simulink model "sevietta_devel_2018a"  (R2013a)
settings: Solver=VariableStepDiscrete  SolverMode=SingleTasking  StartTime=0.0  StopTime=3276  RelTol=1e-3
undefined symbols (not defined in the file): sfp
libraries: xbsIndex_r4 x2589, casper_library_delays x40, simulink x19, casper_library_misc x17, xps_library x13
(part 7 of 32)

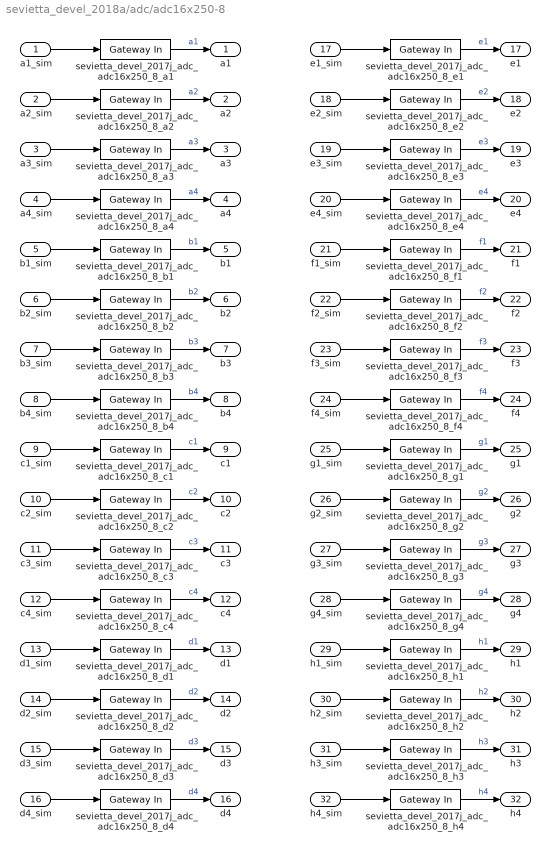
== system sevietta_devel_2018a/adc/adc16x250-8 ==
  a1_sim : Inport
  a2_sim : Inport  Port=2
  a3_sim : Inport  Port=3
  a4_sim : Inport  Port=4
  b1_sim : Inport  Port=5
  b2_sim : Inport  Port=6
  b3_sim : Inport  Port=7
  b4_sim : Inport  Port=8
  c1_sim : Inport  Port=9
  c2_sim : Inport  Port=10
  c3_sim : Inport  Port=11
  c4_sim : Inport  Port=12
  d1_sim : Inport  Port=13
  d2_sim : Inport  Port=14
  d3_sim : Inport  Port=15
  d4_sim : Inport  Port=16
  e1_sim : Inport  Port=17
  e2_sim : Inport  Port=18
  e3_sim : Inport  Port=19
  e4_sim : Inport  Port=20
  f1_sim : Inport  Port=21
  f2_sim : Inport  Port=22
  f3_sim : Inport  Port=23
  f4_sim : Inport  Port=24
  g1_sim : Inport  Port=25
  g2_sim : Inport  Port=26
  g3_sim : Inport  Port=27
  g4_sim : Inport  Port=28
  h1_sim : Inport  Port=29
  h2_sim : Inport  Port=30
  h3_sim : Inport  Port=31
  h4_sim : Inport  Port=32
  sevietta_devel_2017j_adc_adc16x250_8_a{1..4} (4 alike) : xbsIndex_r4/Gateway In  gui_display_data_type=Fixed-point  arith_type="Signed  (2's comp)"  n_bits=8  bin_pt=7  preci_type=Single  exp_width=8  frac_width=24  quantization="Round  (unbiased: +/- Inf)"  overflow=Saturate  period=1  dbl_ovrd=off  timing_constraint=None  locs_specified=off  LOCs={}  UseAsADC=off  ADCChannel='1'  inherit_from_input=off  hdl_port=on  block_type=gatewayin
  sevietta_devel_2017j_adc_adc16x250_8_b{1..4} (4 alike) : xbsIndex_r4/Gateway In  gui_display_data_type=Fixed-point  arith_type="Signed  (2's comp)"  n_bits=8  bin_pt=7  preci_type=Single  exp_width=8  frac_width=24  quantization="Round  (unbiased: +/- Inf)"  overflow=Saturate  period=1  dbl_ovrd=off  timing_constraint=None  locs_specified=off  LOCs={}  UseAsADC=off  ADCChannel='1'  inherit_from_input=off  hdl_port=on  block_type=gatewayin
  sevietta_devel_2017j_adc_adc16x250_8_c{1..4} (4 alike) : xbsIndex_r4/Gateway In  gui_display_data_type=Fixed-point  arith_type="Signed  (2's comp)"  n_bits=8  bin_pt=7  preci_type=Single  exp_width=8  frac_width=24  quantization="Round  (unbiased: +/- Inf)"  overflow=Saturate  period=1  dbl_ovrd=off  timing_constraint=None  locs_specified=off  LOCs={}  UseAsADC=off  ADCChannel='1'  inherit_from_input=off  hdl_port=on  block_type=gatewayin
  sevietta_devel_2017j_adc_adc16x250_8_d{1..4} (4 alike) : xbsIndex_r4/Gateway In  gui_display_data_type=Fixed-point  arith_type="Signed  (2's comp)"  n_bits=8  bin_pt=7  preci_type=Single  exp_width=8  frac_width=24  quantization="Round  (unbiased: +/- Inf)"  overflow=Saturate  period=1  dbl_ovrd=off  timing_constraint=None  locs_specified=off  LOCs={}  UseAsADC=off  ADCChannel='1'  inherit_from_input=off  hdl_port=on  block_type=gatewayin
  sevietta_devel_2017j_adc_adc16x250_8_e{1..4} (4 alike) : xbsIndex_r4/Gateway In  gui_display_data_type=Fixed-point  arith_type="Signed  (2's comp)"  n_bits=8  bin_pt=7  preci_type=Single  exp_width=8  frac_width=24  quantization="Round  (unbiased: +/- Inf)"  overflow=Saturate  period=1  dbl_ovrd=off  timing_constraint=None  locs_specified=off  LOCs={}  UseAsADC=off  ADCChannel='1'  inherit_from_input=off  hdl_port=on  block_type=gatewayin
  sevietta_devel_2017j_adc_adc16x250_8_f{1..4} (4 alike) : xbsIndex_r4/Gateway In  gui_display_data_type=Fixed-point  arith_type="Signed  (2's comp)"  n_bits=8  bin_pt=7  preci_type=Single  exp_width=8  frac_width=24  quantization="Round  (unbiased: +/- Inf)"  overflow=Saturate  period=1  dbl_ovrd=off  timing_constraint=None  locs_specified=off  LOCs={}  UseAsADC=off  ADCChannel='1'  inherit_from_input=off  hdl_port=on  block_type=gatewayin
  sevietta_devel_2017j_adc_adc16x250_8_g{1..4} (4 alike) : xbsIndex_r4/Gateway In  gui_display_data_type=Fixed-point  arith_type="Signed  (2's comp)"  n_bits=8  bin_pt=7  preci_type=Single  exp_width=8  frac_width=24  quantization="Round  (unbiased: +/- Inf)"  overflow=Saturate  period=1  dbl_ovrd=off  timing_constraint=None  locs_specified=off  LOCs={}  UseAsADC=off  ADCChannel='1'  inherit_from_input=off  hdl_port=on  block_type=gatewayin
  sevietta_devel_2017j_adc_adc16x250_8_h{1..4} (4 alike) : xbsIndex_r4/Gateway In  gui_display_data_type=Fixed-point  arith_type="Signed  (2's comp)"  n_bits=8  bin_pt=7  preci_type=Single  exp_width=8  frac_width=24  quantization="Round  (unbiased: +/- Inf)"  overflow=Saturate  period=1  dbl_ovrd=off  timing_constraint=None  locs_specified=off  LOCs={}  UseAsADC=off  ADCChannel='1'  inherit_from_input=off  hdl_port=on  block_type=gatewayin
  a1 : Outport
  a2 : Outport  Port=2
  a3 : Outport  Port=3
  a4 : Outport  Port=4
  b1 : Outport  Port=5
  b2 : Outport  Port=6
  b3 : Outport  Port=7
  b4 : Outport  Port=8
  c1 : Outport  Port=9
  c2 : Outport  Port=10
  c3 : Outport  Port=11
  c4 : Outport  Port=12
  d1 : Outport  Port=13
  d2 : Outport  Port=14
  d3 : Outport  Port=15
  d4 : Outport  Port=16
  e1 : Outport  Port=17
  e2 : Outport  Port=18
  e3 : Outport  Port=19
  e4 : Outport  Port=20
  f1 : Outport  Port=21
  f2 : Outport  Port=22
  f3 : Outport  Port=23
  f4 : Outport  Port=24
  g1 : Outport  Port=25
  g2 : Outport  Port=26
  g3 : Outport  Port=27
  g4 : Outport  Port=28
  h1 : Outport  Port=29
  h2 : Outport  Port=30
  h3 : Outport  Port=31
  h4 : Outport  Port=32
  wires:
  a1_sim/1 -> sevietta_devel_2017j_adc_adc16x250_8_a1/1
  sevietta_devel_2017j_adc_adc16x250_8_a1/1 -> a1/1  "a1"
  a2_sim/1 -> sevietta_devel_2017j_adc_adc16x250_8_a2/1
  sevietta_devel_2017j_adc_adc16x250_8_a2/1 -> a2/1  "a2"
  a3_sim/1 -> sevietta_devel_2017j_adc_adc16x250_8_a3/1
  sevietta_devel_2017j_adc_adc16x250_8_a3/1 -> a3/1  "a3"
  a4_sim/1 -> sevietta_devel_2017j_adc_adc16x250_8_a4/1
  sevietta_devel_2017j_adc_adc16x250_8_a4/1 -> a4/1  "a4"
  b1_sim/1 -> sevietta_devel_2017j_adc_adc16x250_8_b1/1
  sevietta_devel_2017j_adc_adc16x250_8_b1/1 -> b1/1  "b1"
  b2_sim/1 -> sevietta_devel_2017j_adc_adc16x250_8_b2/1
  sevietta_devel_2017j_adc_adc16x250_8_b2/1 -> b2/1  "b2"
  b3_sim/1 -> sevietta_devel_2017j_adc_adc16x250_8_b3/1
  sevietta_devel_2017j_adc_adc16x250_8_b3/1 -> b3/1  "b3"
  b4_sim/1 -> sevietta_devel_2017j_adc_adc16x250_8_b4/1
  sevietta_devel_2017j_adc_adc16x250_8_b4/1 -> b4/1  "b4"
  c1_sim/1 -> sevietta_devel_2017j_adc_adc16x250_8_c1/1
  sevietta_devel_2017j_adc_adc16x250_8_c1/1 -> c1/1  "c1"
  c2_sim/1 -> sevietta_devel_2017j_adc_adc16x250_8_c2/1
  sevietta_devel_2017j_adc_adc16x250_8_c2/1 -> c2/1  "c2"
  c3_sim/1 -> sevietta_devel_2017j_adc_adc16x250_8_c3/1
  sevietta_devel_2017j_adc_adc16x250_8_c3/1 -> c3/1  "c3"
  c4_sim/1 -> sevietta_devel_2017j_adc_adc16x250_8_c4/1
  sevietta_devel_2017j_adc_adc16x250_8_c4/1 -> c4/1  "c4"
  d1_sim/1 -> sevietta_devel_2017j_adc_adc16x250_8_d1/1
  sevietta_devel_2017j_adc_adc16x250_8_d1/1 -> d1/1  "d1"
  d2_sim/1 -> sevietta_devel_2017j_adc_adc16x250_8_d2/1
  sevietta_devel_2017j_adc_adc16x250_8_d2/1 -> d2/1  "d2"
  d3_sim/1 -> sevietta_devel_2017j_adc_adc16x250_8_d3/1
  sevietta_devel_2017j_adc_adc16x250_8_d3/1 -> d3/1  "d3"
  d4_sim/1 -> sevietta_devel_2017j_adc_adc16x250_8_d4/1
  sevietta_devel_2017j_adc_adc16x250_8_d4/1 -> d4/1  "d4"
  e1_sim/1 -> sevietta_devel_2017j_adc_adc16x250_8_e1/1
  sevietta_devel_2017j_adc_adc16x250_8_e1/1 -> e1/1  "e1"
  e2_sim/1 -> sevietta_devel_2017j_adc_adc16x250_8_e2/1
  sevietta_devel_2017j_adc_adc16x250_8_e2/1 -> e2/1  "e2"
  e3_sim/1 -> sevietta_devel_2017j_adc_adc16x250_8_e3/1
  sevietta_devel_2017j_adc_adc16x250_8_e3/1 -> e3/1  "e3"
  e4_sim/1 -> sevietta_devel_2017j_adc_adc16x250_8_e4/1
  sevietta_devel_2017j_adc_adc16x250_8_e4/1 -> e4/1  "e4"
  f1_sim/1 -> sevietta_devel_2017j_adc_adc16x250_8_f1/1
  sevietta_devel_2017j_adc_adc16x250_8_f1/1 -> f1/1  "f1"
  f2_sim/1 -> sevietta_devel_2017j_adc_adc16x250_8_f2/1
  sevietta_devel_2017j_adc_adc16x250_8_f2/1 -> f2/1  "f2"
  f3_sim/1 -> sevietta_devel_2017j_adc_adc16x250_8_f3/1
  sevietta_devel_2017j_adc_adc16x250_8_f3/1 -> f3/1  "f3"
  f4_sim/1 -> sevietta_devel_2017j_adc_adc16x250_8_f4/1
  sevietta_devel_2017j_adc_adc16x250_8_f4/1 -> f4/1  "f4"
  g1_sim/1 -> sevietta_devel_2017j_adc_adc16x250_8_g1/1
  sevietta_devel_2017j_adc_adc16x250_8_g1/1 -> g1/1  "g1"
  g2_sim/1 -> sevietta_devel_2017j_adc_adc16x250_8_g2/1
  sevietta_devel_2017j_adc_adc16x250_8_g2/1 -> g2/1  "g2"
  g3_sim/1 -> sevietta_devel_2017j_adc_adc16x250_8_g3/1
  sevietta_devel_2017j_adc_adc16x250_8_g3/1 -> g3/1  "g3"
  g4_sim/1 -> sevietta_devel_2017j_adc_adc16x250_8_g4/1
  sevietta_devel_2017j_adc_adc16x250_8_g4/1 -> g4/1  "g4"
  h1_sim/1 -> sevietta_devel_2017j_adc_adc16x250_8_h1/1
  sevietta_devel_2017j_adc_adc16x250_8_h1/1 -> h1/1  "h1"
  h2_sim/1 -> sevietta_devel_2017j_adc_adc16x250_8_h2/1
  sevietta_devel_2017j_adc_adc16x250_8_h2/1 -> h2/1  "h2"
  h3_sim/1 -> sevietta_devel_2017j_adc_adc16x250_8_h3/1
  sevietta_devel_2017j_adc_adc16x250_8_h3/1 -> h3/1  "h3"
  h4_sim/1 -> sevietta_devel_2017j_adc_adc16x250_8_h4/1
  sevietta_devel_2017j_adc_adc16x250_8_h4/1 -> h4/1  "h4"

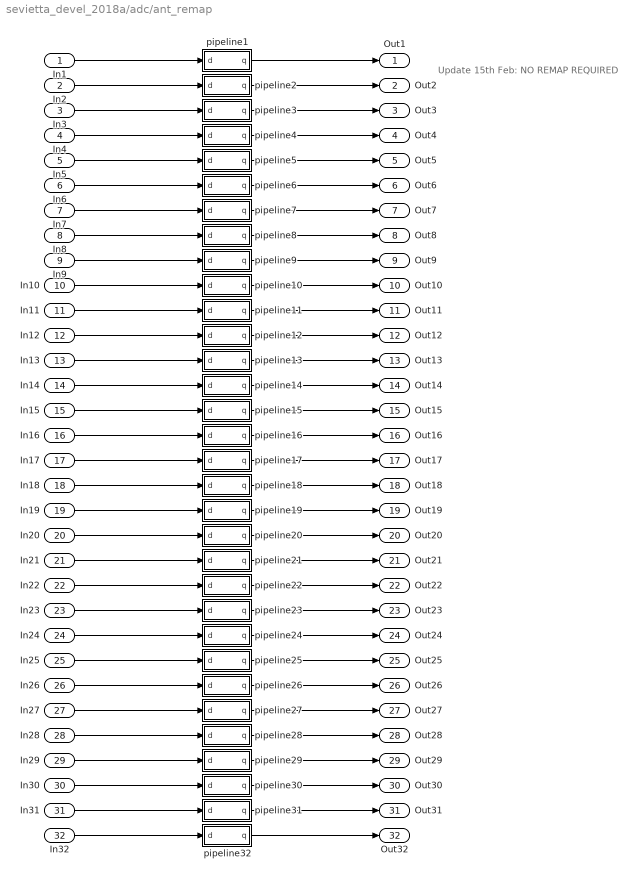
== system sevietta_devel_2018a/adc/ant_remap ==
  note: Update 15th Feb: NO REMAP REQUIRED
  In1 : Inport
  In2 : Inport  Port=2
  In3 : Inport  Port=3
  In4 : Inport  Port=4
  In5 : Inport  Port=5
  In6 : Inport  Port=6
  In7 : Inport  Port=7
  In8 : Inport  Port=8
  In9 : Inport  Port=9
  In10 : Inport  Port=10
  In11 : Inport  Port=11
  In12 : Inport  Port=12
  In13 : Inport  Port=13
  In14 : Inport  Port=14
  In15 : Inport  Port=15
  In16 : Inport  Port=16
  In17 : Inport  Port=17
  In18 : Inport  Port=18
  In19 : Inport  Port=19
  In20 : Inport  Port=20
  In21 : Inport  Port=21
  In22 : Inport  Port=22
  In23 : Inport  Port=23
  In24 : Inport  Port=24
  In25 : Inport  Port=25
  In26 : Inport  Port=26
  In27 : Inport  Port=27
  In28 : Inport  Port=28
  In29 : Inport  Port=29
  In30 : Inport  Port=30
  In31 : Inport  Port=31
  In32 : Inport  Port=32
  pipeline1 : Subsystem  AncestorBlock=casper_library_delays/pipeline  mask(pipeline){latency=1}
      mask help:
      | An explicitly laid-out delay line to avoid mapping to SRL16s
      | for use in pipelining to help achieve timing closure.
      mask init:
      | pipeline_init(gcb,'latency',latency);
      settings: AttributesFormatString=Latency = %<latency>
      mask Display:
      | port_label('input', 1, 'd');
      | port_label('output', 1, 'q');
      | disp(['Z^-', num2str(latency)]);
  pipeline10 : Subsystem  AncestorBlock=casper_library_delays/pipeline  mask(pipeline){latency=1}
      mask help:
      | An explicitly laid-out delay line to avoid mapping to SRL16s
      | for use in pipelining to help achieve timing closure.
      mask init:
      | pipeline_init(gcb,'latency',latency);
      settings: AttributesFormatString=Latency = %<latency>
      mask Display:
      | port_label('input', 1, 'd');
      | port_label('output', 1, 'q');
      | disp(['Z^-', num2str(latency)]);
  pipeline11 : Subsystem  AncestorBlock=casper_library_delays/pipeline  mask(pipeline){latency=1}
      mask help:
      | An explicitly laid-out delay line to avoid mapping to SRL16s
      | for use in pipelining to help achieve timing closure.
      mask init:
      | pipeline_init(gcb,'latency',latency);
      settings: AttributesFormatString=Latency = %<latency>
      mask Display:
      | port_label('input', 1, 'd');
      | port_label('output', 1, 'q');
      | disp(['Z^-', num2str(latency)]);
  pipeline12 : Subsystem  AncestorBlock=casper_library_delays/pipeline  mask(pipeline){latency=1}
      mask help:
      | An explicitly laid-out delay line to avoid mapping to SRL16s
      | for use in pipelining to help achieve timing closure.
      mask init:
      | pipeline_init(gcb,'latency',latency);
      settings: AttributesFormatString=Latency = %<latency>
      mask Display:
      | port_label('input', 1, 'd');
      | port_label('output', 1, 'q');
      | disp(['Z^-', num2str(latency)]);
  pipeline13 : Subsystem  AncestorBlock=casper_library_delays/pipeline  mask(pipeline){latency=1}
      mask help:
      | An explicitly laid-out delay line to avoid mapping to SRL16s
      | for use in pipelining to help achieve timing closure.
      mask init:
      | pipeline_init(gcb,'latency',latency);
      settings: AttributesFormatString=Latency = %<latency>
      mask Display:
      | port_label('input', 1, 'd');
      | port_label('output', 1, 'q');
      | disp(['Z^-', num2str(latency)]);
  pipeline14 : Subsystem  AncestorBlock=casper_library_delays/pipeline  mask(pipeline){latency=1}
      mask help:
      | An explicitly laid-out delay line to avoid mapping to SRL16s
      | for use in pipelining to help achieve timing closure.
      mask init:
      | pipeline_init(gcb,'latency',latency);
      settings: AttributesFormatString=Latency = %<latency>
      mask Display:
      | port_label('input', 1, 'd');
      | port_label('output', 1, 'q');
      | disp(['Z^-', num2str(latency)]);
  pipeline15 : Subsystem  AncestorBlock=casper_library_delays/pipeline  mask(pipeline){latency=1}
      mask help:
      | An explicitly laid-out delay line to avoid mapping to SRL16s
      | for use in pipelining to help achieve timing closure.
      mask init:
      | pipeline_init(gcb,'latency',latency);
      settings: AttributesFormatString=Latency = %<latency>
      mask Display:
      | port_label('input', 1, 'd');
      | port_label('output', 1, 'q');
      | disp(['Z^-', num2str(latency)]);
  pipeline16 : Subsystem  AncestorBlock=casper_library_delays/pipeline  mask(pipeline){latency=1}
      mask help:
      | An explicitly laid-out delay line to avoid mapping to SRL16s
      | for use in pipelining to help achieve timing closure.
      mask init:
      | pipeline_init(gcb,'latency',latency);
      settings: AttributesFormatString=Latency = %<latency>
      mask Display:
      | port_label('input', 1, 'd');
      | port_label('output', 1, 'q');
      | disp(['Z^-', num2str(latency)]);
  pipeline17 : Subsystem  AncestorBlock=casper_library_delays/pipeline  mask(pipeline){latency=1}
      mask help:
      | An explicitly laid-out delay line to avoid mapping to SRL16s
      | for use in pipelining to help achieve timing closure.
      mask init:
      | pipeline_init(gcb,'latency',latency);
      settings: AttributesFormatString=Latency = %<latency>
      mask Display:
      | port_label('input', 1, 'd');
      | port_label('output', 1, 'q');
      | disp(['Z^-', num2str(latency)]);
  pipeline18 : Subsystem  AncestorBlock=casper_library_delays/pipeline  mask(pipeline){latency=1}
      mask help:
      | An explicitly laid-out delay line to avoid mapping to SRL16s
      | for use in pipelining to help achieve timing closure.
      mask init:
      | pipeline_init(gcb,'latency',latency);
      settings: AttributesFormatString=Latency = %<latency>
      mask Display:
      | port_label('input', 1, 'd');
      | port_label('output', 1, 'q');
      | disp(['Z^-', num2str(latency)]);
  pipeline19 : Subsystem  AncestorBlock=casper_library_delays/pipeline  mask(pipeline){latency=1}
      mask help:
      | An explicitly laid-out delay line to avoid mapping to SRL16s
      | for use in pipelining to help achieve timing closure.
      mask init:
      | pipeline_init(gcb,'latency',latency);
      settings: AttributesFormatString=Latency = %<latency>
      mask Display:
      | port_label('input', 1, 'd');
      | port_label('output', 1, 'q');
      | disp(['Z^-', num2str(latency)]);
  pipeline2 : Subsystem  AncestorBlock=casper_library_delays/pipeline  mask(pipeline){latency=1}
      mask help:
      | An explicitly laid-out delay line to avoid mapping to SRL16s
      | for use in pipelining to help achieve timing closure.
      mask init:
      | pipeline_init(gcb,'latency',latency);
      settings: AttributesFormatString=Latency = %<latency>
      mask Display:
      | port_label('input', 1, 'd');
      | port_label('output', 1, 'q');
      | disp(['Z^-', num2str(latency)]);
  pipeline20 : Subsystem  AncestorBlock=casper_library_delays/pipeline  mask(pipeline){latency=1}
      mask help:
      | An explicitly laid-out delay line to avoid mapping to SRL16s
      | for use in pipelining to help achieve timing closure.
      mask init:
      | pipeline_init(gcb,'latency',latency);
      settings: AttributesFormatString=Latency = %<latency>
      mask Display:
      | port_label('input', 1, 'd');
      | port_label('output', 1, 'q');
      | disp(['Z^-', num2str(latency)]);
  pipeline21 : Subsystem  AncestorBlock=casper_library_delays/pipeline  mask(pipeline){latency=1}
      mask help:
      | An explicitly laid-out delay line to avoid mapping to SRL16s
      | for use in pipelining to help achieve timing closure.
      mask init:
      | pipeline_init(gcb,'latency',latency);
      settings: AttributesFormatString=Latency = %<latency>
      mask Display:
      | port_label('input', 1, 'd');
      | port_label('output', 1, 'q');
      | disp(['Z^-', num2str(latency)]);
  pipeline22 : Subsystem  AncestorBlock=casper_library_delays/pipeline  mask(pipeline){latency=1}
      mask help:
      | An explicitly laid-out delay line to avoid mapping to SRL16s
      | for use in pipelining to help achieve timing closure.
      mask init:
      | pipeline_init(gcb,'latency',latency);
      settings: AttributesFormatString=Latency = %<latency>
      mask Display:
      | port_label('input', 1, 'd');
      | port_label('output', 1, 'q');
      | disp(['Z^-', num2str(latency)]);
  pipeline23 : Subsystem  AncestorBlock=casper_library_delays/pipeline  mask(pipeline){latency=1}
      mask help:
      | An explicitly laid-out delay line to avoid mapping to SRL16s
      | for use in pipelining to help achieve timing closure.
      mask init:
      | pipeline_init(gcb,'latency',latency);
      settings: AttributesFormatString=Latency = %<latency>
      mask Display:
      | port_label('input', 1, 'd');
      | port_label('output', 1, 'q');
      | disp(['Z^-', num2str(latency)]);
  pipeline24 : Subsystem  AncestorBlock=casper_library_delays/pipeline  mask(pipeline){latency=1}
      mask help:
      | An explicitly laid-out delay line to avoid mapping to SRL16s
      | for use in pipelining to help achieve timing closure.
      mask init:
      | pipeline_init(gcb,'latency',latency);
      settings: AttributesFormatString=Latency = %<latency>
      mask Display:
      | port_label('input', 1, 'd');
      | port_label('output', 1, 'q');
      | disp(['Z^-', num2str(latency)]);
  pipeline25 : Subsystem  AncestorBlock=casper_library_delays/pipeline  mask(pipeline){latency=1}
      mask help:
      | An explicitly laid-out delay line to avoid mapping to SRL16s
      | for use in pipelining to help achieve timing closure.
      mask init:
      | pipeline_init(gcb,'latency',latency);
      settings: AttributesFormatString=Latency = %<latency>
      mask Display:
      | port_label('input', 1, 'd');
      | port_label('output', 1, 'q');
      | disp(['Z^-', num2str(latency)]);
  pipeline26 : Subsystem  AncestorBlock=casper_library_delays/pipeline  mask(pipeline){latency=1}
      mask help:
      | An explicitly laid-out delay line to avoid mapping to SRL16s
      | for use in pipelining to help achieve timing closure.
      mask init:
      | pipeline_init(gcb,'latency',latency);
      settings: AttributesFormatString=Latency = %<latency>
      mask Display:
      | port_label('input', 1, 'd');
      | port_label('output', 1, 'q');
      | disp(['Z^-', num2str(latency)]);
  pipeline27 : Subsystem  AncestorBlock=casper_library_delays/pipeline  mask(pipeline){latency=1}
      mask help:
      | An explicitly laid-out delay line to avoid mapping to SRL16s
      | for use in pipelining to help achieve timing closure.
      mask init:
      | pipeline_init(gcb,'latency',latency);
      settings: AttributesFormatString=Latency = %<latency>
      mask Display:
      | port_label('input', 1, 'd');
      | port_label('output', 1, 'q');
      | disp(['Z^-', num2str(latency)]);
  pipeline28 : Subsystem  AncestorBlock=casper_library_delays/pipeline  mask(pipeline){latency=1}
      mask help:
      | An explicitly laid-out delay line to avoid mapping to SRL16s
      | for use in pipelining to help achieve timing closure.
      mask init:
      | pipeline_init(gcb,'latency',latency);
      settings: AttributesFormatString=Latency = %<latency>
      mask Display:
      | port_label('input', 1, 'd');
      | port_label('output', 1, 'q');
      | disp(['Z^-', num2str(latency)]);
  pipeline29 : Subsystem  AncestorBlock=casper_library_delays/pipeline  mask(pipeline){latency=1}
      mask help:
      | An explicitly laid-out delay line to avoid mapping to SRL16s
      | for use in pipelining to help achieve timing closure.
      mask init:
      | pipeline_init(gcb,'latency',latency);
      settings: AttributesFormatString=Latency = %<latency>
      mask Display:
      | port_label('input', 1, 'd');
      | port_label('output', 1, 'q');
      | disp(['Z^-', num2str(latency)]);
  pipeline3 : Subsystem  AncestorBlock=casper_library_delays/pipeline  mask(pipeline){latency=1}
      mask help:
      | An explicitly laid-out delay line to avoid mapping to SRL16s
      | for use in pipelining to help achieve timing closure.
      mask init:
      | pipeline_init(gcb,'latency',latency);
      settings: AttributesFormatString=Latency = %<latency>
      mask Display:
      | port_label('input', 1, 'd');
      | port_label('output', 1, 'q');
      | disp(['Z^-', num2str(latency)]);
  pipeline30 : Subsystem  AncestorBlock=casper_library_delays/pipeline  mask(pipeline){latency=1}
      mask help:
      | An explicitly laid-out delay line to avoid mapping to SRL16s
      | for use in pipelining to help achieve timing closure.
      mask init:
      | pipeline_init(gcb,'latency',latency);
      settings: AttributesFormatString=Latency = %<latency>
      mask Display:
      | port_label('input', 1, 'd');
      | port_label('output', 1, 'q');
      | disp(['Z^-', num2str(latency)]);
  pipeline31 : Subsystem  AncestorBlock=casper_library_delays/pipeline  mask(pipeline){latency=1}
      mask help:
      | An explicitly laid-out delay line to avoid mapping to SRL16s
      | for use in pipelining to help achieve timing closure.
      mask init:
      | pipeline_init(gcb,'latency',latency);
      settings: AttributesFormatString=Latency = %<latency>
      mask Display:
      | port_label('input', 1, 'd');
      | port_label('output', 1, 'q');
      | disp(['Z^-', num2str(latency)]);
  pipeline32 : Subsystem  AncestorBlock=casper_library_delays/pipeline  mask(pipeline){latency=1}
      mask help:
      | An explicitly laid-out delay line to avoid mapping to SRL16s
      | for use in pipelining to help achieve timing closure.
      mask init:
      | pipeline_init(gcb,'latency',latency);
      settings: AttributesFormatString=Latency = %<latency>
      mask Display:
      | port_label('input', 1, 'd');
      | port_label('output', 1, 'q');
      | disp(['Z^-', num2str(latency)]);
  pipeline4 : Subsystem  AncestorBlock=casper_library_delays/pipeline  mask(pipeline){latency=1}
      mask help:
      | An explicitly laid-out delay line to avoid mapping to SRL16s
      | for use in pipelining to help achieve timing closure.
      mask init:
      | pipeline_init(gcb,'latency',latency);
      settings: AttributesFormatString=Latency = %<latency>
      mask Display:
      | port_label('input', 1, 'd');
      | port_label('output', 1, 'q');
      | disp(['Z^-', num2str(latency)]);
  pipeline5 : Subsystem  AncestorBlock=casper_library_delays/pipeline  mask(pipeline){latency=1}
      mask help:
      | An explicitly laid-out delay line to avoid mapping to SRL16s
      | for use in pipelining to help achieve timing closure.
      mask init:
      | pipeline_init(gcb,'latency',latency);
      settings: AttributesFormatString=Latency = %<latency>
      mask Display:
      | port_label('input', 1, 'd');
      | port_label('output', 1, 'q');
      | disp(['Z^-', num2str(latency)]);
  pipeline6 : Subsystem  AncestorBlock=casper_library_delays/pipeline  mask(pipeline){latency=1}
      mask help:
      | An explicitly laid-out delay line to avoid mapping to SRL16s
      | for use in pipelining to help achieve timing closure.
      mask init:
      | pipeline_init(gcb,'latency',latency);
      settings: AttributesFormatString=Latency = %<latency>
      mask Display:
      | port_label('input', 1, 'd');
      | port_label('output', 1, 'q');
      | disp(['Z^-', num2str(latency)]);
  pipeline7 : Subsystem  AncestorBlock=casper_library_delays/pipeline  mask(pipeline){latency=1}
      mask help:
      | An explicitly laid-out delay line to avoid mapping to SRL16s
      | for use in pipelining to help achieve timing closure.
      mask init:
      | pipeline_init(gcb,'latency',latency);
      settings: AttributesFormatString=Latency = %<latency>
      mask Display:
      | port_label('input', 1, 'd');
      | port_label('output', 1, 'q');
      | disp(['Z^-', num2str(latency)]);
  pipeline8 : Subsystem  AncestorBlock=casper_library_delays/pipeline  mask(pipeline){latency=1}
      mask help:
      | An explicitly laid-out delay line to avoid mapping to SRL16s
      | for use in pipelining to help achieve timing closure.
      mask init:
      | pipeline_init(gcb,'latency',latency);
      settings: AttributesFormatString=Latency = %<latency>
      mask Display:
      | port_label('input', 1, 'd');
      | port_label('output', 1, 'q');
      | disp(['Z^-', num2str(latency)]);
  pipeline9 : Subsystem  AncestorBlock=casper_library_delays/pipeline  mask(pipeline){latency=1}
      mask help:
      | An explicitly laid-out delay line to avoid mapping to SRL16s
      | for use in pipelining to help achieve timing closure.
      mask init:
      | pipeline_init(gcb,'latency',latency);
      settings: AttributesFormatString=Latency = %<latency>
      mask Display:
      | port_label('input', 1, 'd');
      | port_label('output', 1, 'q');
      | disp(['Z^-', num2str(latency)]);
  Out1 : Outport
  Out2 : Outport  Port=2
  Out3 : Outport  Port=3
  Out4 : Outport  Port=4
  Out5 : Outport  Port=5
  Out6 : Outport  Port=6
  Out7 : Outport  Port=7
  Out8 : Outport  Port=8
  Out9 : Outport  Port=9
  Out10 : Outport  Port=10
  Out11 : Outport  Port=11
  Out12 : Outport  Port=12
  Out13 : Outport  Port=13
  Out14 : Outport  Port=14
  Out15 : Outport  Port=15
  Out16 : Outport  Port=16
  Out17 : Outport  Port=17
  Out18 : Outport  Port=18
  Out19 : Outport  Port=19
  Out20 : Outport  Port=20
  Out21 : Outport  Port=21
  Out22 : Outport  Port=22
  Out23 : Outport  Port=23
  Out24 : Outport  Port=24
  Out25 : Outport  Port=25
  Out26 : Outport  Port=26
  Out27 : Outport  Port=27
  Out28 : Outport  Port=28
  Out29 : Outport  Port=29
  Out30 : Outport  Port=30
  Out31 : Outport  Port=31
  Out32 : Outport  Port=32
  wires:
  In1/1 -> pipeline1/1(d)
  In2/1 -> pipeline2/1(d)
  In3/1 -> pipeline3/1(d)
  In4/1 -> pipeline4/1(d)
  In5/1 -> pipeline5/1(d)
  In6/1 -> pipeline6/1(d)
  In7/1 -> pipeline7/1(d)
  In8/1 -> pipeline8/1(d)
  In9/1 -> pipeline9/1(d)
  In10/1 -> pipeline10/1(d)
  In11/1 -> pipeline11/1(d)
  In12/1 -> pipeline12/1(d)
  In13/1 -> pipeline13/1(d)
  In14/1 -> pipeline14/1(d)
  In15/1 -> pipeline15/1(d)
  In16/1 -> pipeline16/1(d)
  In17/1 -> pipeline17/1(d)
  In18/1 -> pipeline18/1(d)
  In19/1 -> pipeline19/1(d)
  In20/1 -> pipeline20/1(d)
  In21/1 -> pipeline21/1(d)
  In22/1 -> pipeline22/1(d)
  In23/1 -> pipeline23/1(d)
  In24/1 -> pipeline24/1(d)
  In25/1 -> pipeline25/1(d)
  In26/1 -> pipeline26/1(d)
  In27/1 -> pipeline27/1(d)
  In28/1 -> pipeline28/1(d)
  In29/1 -> pipeline29/1(d)
  In30/1 -> pipeline30/1(d)
  In31/1 -> pipeline31/1(d)
  In32/1 -> pipeline32/1(d)
  pipeline1/1(q) -> Out1/1
  pipeline2/1(q) -> Out2/1
  pipeline3/1(q) -> Out3/1
  pipeline4/1(q) -> Out4/1
  pipeline5/1(q) -> Out5/1
  pipeline6/1(q) -> Out6/1
  pipeline7/1(q) -> Out7/1
  pipeline8/1(q) -> Out8/1
  pipeline9/1(q) -> Out9/1
  pipeline10/1(q) -> Out10/1
  pipeline11/1(q) -> Out11/1
  pipeline12/1(q) -> Out12/1
  pipeline13/1(q) -> Out13/1
  pipeline14/1(q) -> Out14/1
  pipeline15/1(q) -> Out15/1
  pipeline16/1(q) -> Out16/1
  pipeline17/1(q) -> Out17/1
  pipeline18/1(q) -> Out18/1
  pipeline19/1(q) -> Out19/1
  pipeline20/1(q) -> Out20/1
  pipeline21/1(q) -> Out21/1
  pipeline22/1(q) -> Out22/1
  pipeline23/1(q) -> Out23/1
  pipeline24/1(q) -> Out24/1
  pipeline25/1(q) -> Out25/1
  pipeline26/1(q) -> Out26/1
  pipeline27/1(q) -> Out27/1
  pipeline28/1(q) -> Out28/1
  pipeline29/1(q) -> Out29/1
  pipeline30/1(q) -> Out30/1
  pipeline31/1(q) -> Out31/1
  pipeline32/1(q) -> Out32/1
